simulink model "harness"  (R2023a)
settings: Solver=VariableStepAuto  StartTime=0.0  StopTime=90  FixedStep=0.001  RelTol=1e-3  EnableMultiTasking=on
model workspace (MAT data in the model file):
  c = Simulink.Parameter
  c.Value = 1500
  c.DataType = 'double'
  c.DocUnits = 'Ns/m'
  c.Complexity = 'real'
  c.Dimensions = [1 1]
  k1 = Simulink.Parameter
  k1.Value = 29000
  k1.DataType = 'double'
  k1.DocUnits = 'N/m'
  k1.Complexity = 'real'
  k1.Dimensions = [1 1]
  k2 = Simulink.Parameter
  k2.Value = 228000
  k2.DataType = 'double'
  k2.DocUnits = 'N/m'
  k2.Complexity = 'real'
  k2.Dimensions = [1 1]
  m1 = Simulink.Parameter
  m1.Value = 380
  m1.DataType = 'double'
  m1.DocUnits = 'kg'
  m1.Complexity = 'real'
  m1.Dimensions = [1 1]
  m2 = Simulink.Parameter
  m2.Value = 31
  m2.DataType = 'double'
  m2.DocUnits = 'kg'
  m2.Complexity = 'real'
  m2.Dimensions = [1 1]
undefined symbols (not defined in the file): DiscIntNeverNeededParam
libraries: simulink x2
settings Model: Creator=david  LastModifiedBy=david
settings DebuggingCC: UnconnectedInputMsg=warning  UnconnectedOutputMsg=warning  UnconnectedLineMsg=warning
settings ModelReferenceCC: EnableRefExpFcnMdlSchedulingChecks=on
settings RTWCC: DLArmComputeVersion=19.05
settings ConfigComp: CovMetricSettings=dcwe

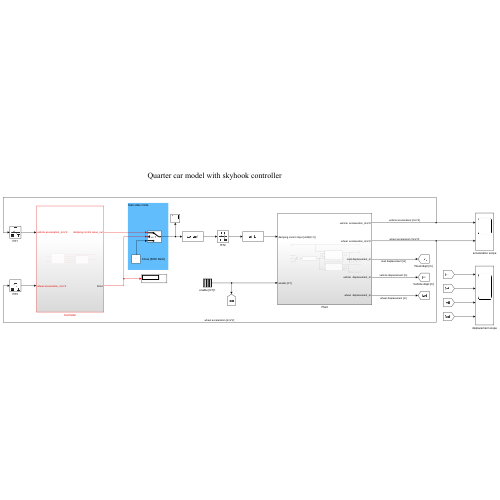
[thumbnail: Simulink's stored preview of the top-level diagram]
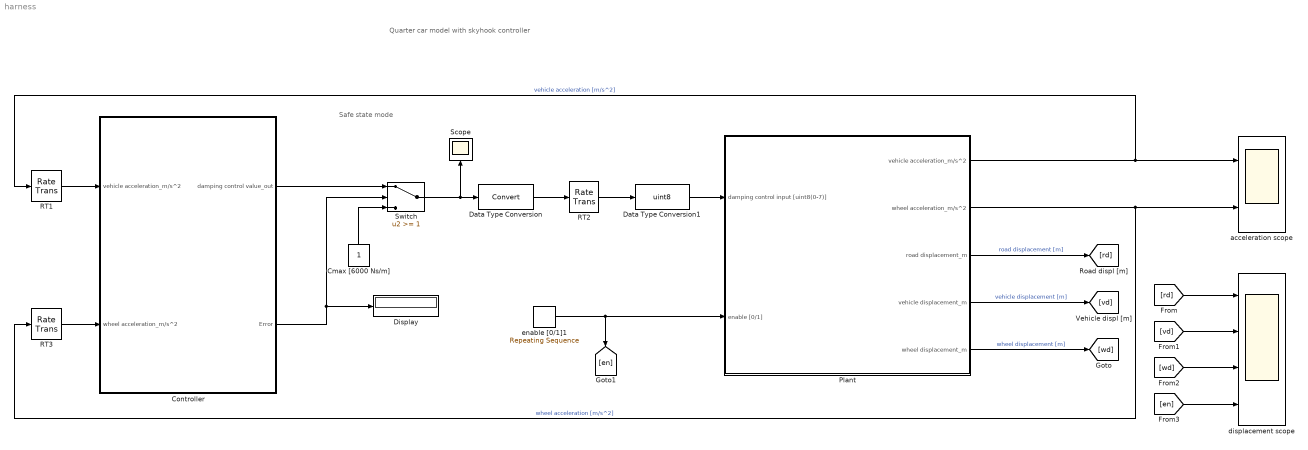
== system harness ==
  note: Safe state mode
  note: Quarter car model with skyhook controller
  Cmax [6000 Ns/m] : Constant  OutDataTypeStr=uint8
  Controller : Subsystem
  Data Type Conversion : DataTypeConversion  SaturateOnIntegerOverflow=off  RndMeth=Floor
  Data Type Conversion1 : DataTypeConversion  OutDataTypeStr=uint8  SaturateOnIntegerOverflow=off  RndMeth=Floor
  Display : Display
  Plant : Subsystem
  RT1 : RateTransition
  RT2 : RateTransition
  RT3 : RateTransition
  Scope : Scope
  Switch : Switch  Threshold=1  SaturateOnIntegerOverflow=off  InputSameDT=off
  acceleration scope : Scope  NumInputPorts=2
  displacement scope : Scope  NumInputPorts=4
  enable [0/1]1 : simulink/Sources/Repeating Sequence  rep_seq_t="[0 10  20 20.1 40 50 80 80.1]"  rep_seq_y=[0 0 0 1 1 1 1 1]
  wires:
  RT2/1 -> Data Type Conversion1/1
  Data Type Conversion1/1 -> Plant/1("damping control input [uint8(0-7)] ")
  Data Type Conversion/1 -> RT2/1
  enable [0/1]1/1 -> Plant/2(enable [0/1]), [en]
  Plant/4(vehicle displacement_m) -> [vd]  "vehicle displacement [m]"
  [wd] -> displacement scope/3
  [en] -> displacement scope/4
  Plant/5(wheel displacement_m) -> [wd]  "wheel displacement [m]"
  [rd] -> displacement scope/1
  Plant/1(vehicle acceleration_m/s^2) -> RT1/1, acceleration scope/1  "vehicle acceleration [m/s^2]"
  Plant/3(road displacement_m) -> [rd]  "road displacement [m]"
  [vd] -> displacement scope/2
  Plant/2(wheel acceleration_m/s^2) -> acceleration scope/2, RT3/1  "wheel acceleration [m/s^2]"
  Controller/1(damping control value_out) -> Switch/1
  RT1/1 -> Controller/1(vehicle acceleration_m/s^2)
  RT3/1 -> Controller/2(wheel acceleration_m/s^2)
  Controller/2(Error) -> Switch/2, Display/1
  Cmax [6000 Ns/m]/1 -> Switch/3
  Switch/1 -> Data Type Conversion/1, Scope/1

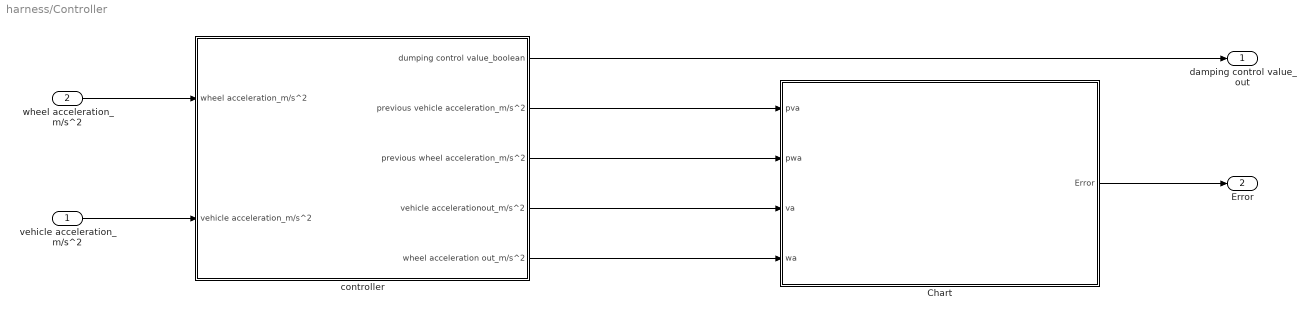
== system harness/Controller ==
  vehicle acceleration_m/s^2 : Inport  OutDataTypeStr=double  Unit=m/s^2  PortDimensions=1
  wheel acceleration_m/s^2 : Inport  Port=2  OutDataTypeStr=double  Unit=m/s^2  PortDimensions=1
  Chart : Stateflow chart  TreatAsAtomicUnit=on
  controller : Subsystem
  damping control value_out : Outport  OutDataTypeStr=uint8  PortDimensions=1  VectorParamsAs1DForOutWhenUnconnected=off
  Error : Outport  Port=2
  wires:
  vehicle acceleration_m/s^2/1 -> controller/2(vehicle acceleration_m/s^2)
  wheel acceleration_m/s^2/1 -> controller/1(wheel acceleration_m/s^2)
  Chart/1(Error) -> Error/1
  controller/1(dumping control value_boolean) -> damping control value_out/1
  controller/2(previous vehicle acceleration_m/s^2) -> Chart/1(pva)
  controller/3(previous wheel acceleration_m/s^2) -> Chart/2(pwa)
  controller/4(vehicle accelerationout_m/s^2) -> Chart/3(va)
  controller/5(wheel acceleration out_m/s^2) -> Chart/4(wa)

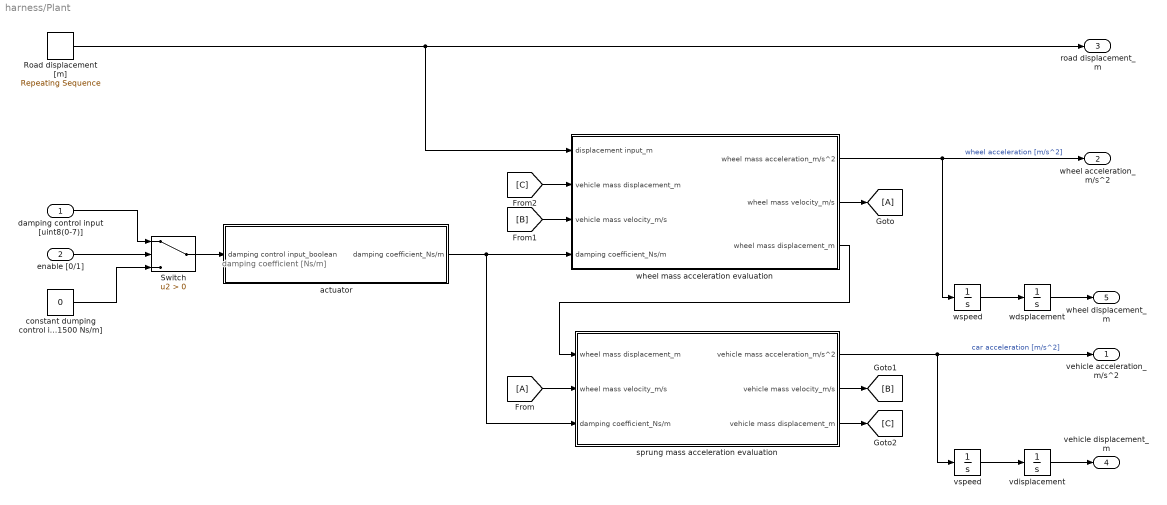
== system harness/Plant ==
  note: damping coefficient [Ns/m]
  "damping control input [uint8(0-7)] " : Inport  OutDataTypeStr=uint8
  enable [0/1] : Inport  Port=2
  From : From
  Goto : Goto
  Road displacement [m] : simulink/Sources/Repeating Sequence  rep_seq_t=[0 0.1 4 4.1 8 10 10.1 10.2 10.3 14]  rep_seq_y=[0 0.2 -0.2 0 -0.2 0 0.2 0.2 0 0]
  Switch : Switch  Criteria=u2 > Threshold  SaturateOnIntegerOverflow=off  InputSameDT=off
  actuator : Subsystem
  constant dumping control input [0=1500 Ns/m] : Constant  Value=0
  sprung mass acceleration evaluation : Subsystem
  vdisplacement : Integrator
  vspeed : Integrator
  wdsplacement : Integrator
  wheel mass acceleration evaluation : Subsystem
  wspeed : Integrator
  vehicle acceleration_m/s^2 : Outport  VectorParamsAs1DForOutWhenUnconnected=off
  wheel acceleration_m/s^2 : Outport  Port=2  Unit=m/s^2  VectorParamsAs1DForOutWhenUnconnected=off
  road displacement_m : Outport  Port=3  Unit=m  VectorParamsAs1DForOutWhenUnconnected=off
  vehicle displacement_m : Outport  Port=4  Unit=m  VectorParamsAs1DForOutWhenUnconnected=off
  wheel displacement_m : Outport  Port=5  Unit=m  VectorParamsAs1DForOutWhenUnconnected=off
  wires:
  Switch/1 -> actuator/1("damping control input_boolean ")
  actuator/1(damping coefficient_Ns/m) -> sprung mass acceleration evaluation/3(damping coefficient_Ns/m), wheel mass acceleration evaluation/4(damping coefficient_Ns/m)
  wheel mass acceleration evaluation/1(wheel mass acceleration_m/s^2) -> wheel acceleration_m/s^2/1, wspeed/1  "wheel acceleration [m/s^2]"
  wheel mass acceleration evaluation/2(wheel mass velocity_m/s) -> Goto/1
  sprung mass acceleration evaluation/1(vehicle mass acceleration_m/s^2) -> vehicle acceleration_m/s^2/1, vspeed/1  "car acceleration [m/s^2]"
  sprung mass acceleration evaluation/2(vehicle mass velocity_m/s) -> [B]
  enable [0/1]/1 -> Switch/2
  wspeed/1 -> wdsplacement/1
  From/1 -> sprung mass acceleration evaluation/2(wheel mass velocity_m/s)
  vspeed/1 -> vdisplacement/1
  wdsplacement/1 -> wheel displacement_m/1
  constant dumping control input [0=1500 Ns/m]/1 -> Switch/3
  Road displacement [m]/1 -> road displacement_m/1, wheel mass acceleration evaluation/1(displacement input_m)
  wheel mass acceleration evaluation/3(wheel mass displacement_m) -> sprung mass acceleration evaluation/1(wheel mass displacement_m)
  "damping control input [uint8(0-7)] "/1 -> Switch/1
  vdisplacement/1 -> vehicle displacement_m/1
  [B] -> wheel mass acceleration evaluation/3(vehicle mass velocity_m/s)
  sprung mass acceleration evaluation/3(vehicle mass displacement_m) -> [C]
  [C] -> wheel mass acceleration evaluation/2(vehicle mass displacement_m)

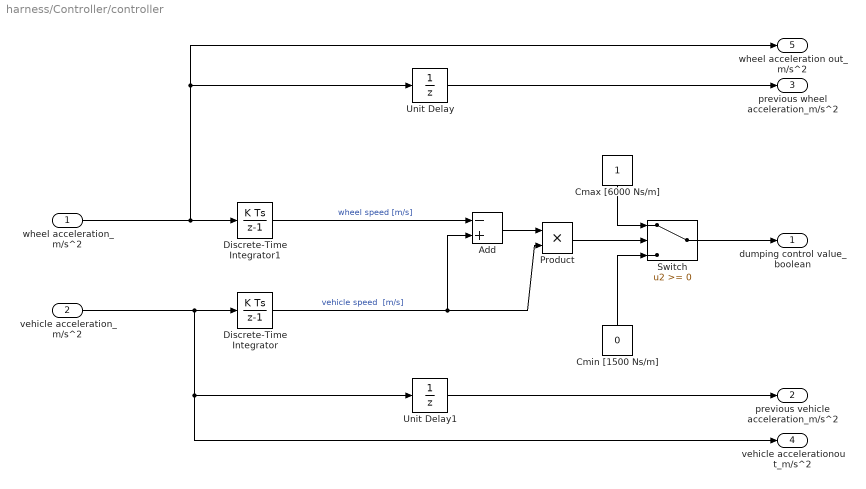
== system harness/Controller/controller ==
  wheel acceleration_m/s^2 : Inport
  vehicle acceleration_m/s^2 : Inport  Port=2  OutDataTypeStr=double  PortDimensions=1
  Add : Sum  Inputs=-+
  Cmax [6000 Ns/m] : Constant  OutDataTypeStr=uint8
  Cmin [1500 Ns/m] : Constant  Value=0  OutDataTypeStr=uint8
  Discrete-Time Integrator : DiscreteIntegrator  SampleTime=-1  ICPrevOutput=DiscIntNeverNeededParam  ICPrevScaledInput=DiscIntNeverNeededParam
  Discrete-Time Integrator1 : DiscreteIntegrator  SampleTime=-1  ICPrevOutput=DiscIntNeverNeededParam  ICPrevScaledInput=DiscIntNeverNeededParam
  Product : Product
  Switch : Switch  SaturateOnIntegerOverflow=off  InputSameDT=off
  Unit Delay : UnitDelay  SampleTime=-1  HasFrameUpgradeWarning=on
  Unit Delay1 : UnitDelay  SampleTime=-1  HasFrameUpgradeWarning=on
  dumping control value_boolean : Outport  OutDataTypeStr=uint8  VectorParamsAs1DForOutWhenUnconnected=off
  previous vehicle acceleration_m/s^2 : Outport  Port=2
  previous wheel acceleration_m/s^2 : Outport  Port=3
  vehicle accelerationout_m/s^2 : Outport  Port=4
  wheel acceleration out_m/s^2 : Outport  Port=5
  wires:
  wheel acceleration_m/s^2/1 -> wheel acceleration out_m/s^2/1, Unit Delay/1, Discrete-Time Integrator1/1
  Cmax [6000 Ns/m]/1 -> Switch/1
  Cmin [1500 Ns/m]/1 -> Switch/3
  Discrete-Time Integrator/1 -> Product/2, Add/2  "vehicle speed  [m/s]"
  Add/1 -> Product/1
  vehicle acceleration_m/s^2/1 -> vehicle accelerationout_m/s^2/1, Unit Delay1/1, Discrete-Time Integrator/1
  Product/1 -> Switch/2
  Discrete-Time Integrator1/1 -> Add/1  "wheel speed [m/s]"
  Unit Delay/1 -> previous wheel acceleration_m/s^2/1
  Unit Delay1/1 -> previous vehicle acceleration_m/s^2/1
  Switch/1 -> dumping control value_boolean/1

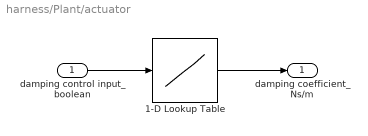
== system harness/Plant/actuator ==
  "damping control input_boolean " : Inport
  1-D Lookup Table : Lookup_n-D  NumberOfTableDimensions=1  BreakpointsForDimension1=uint8([0,1]);  Table=[1500,6000]  InternalRulePriority=Speed  RndMeth=Simplest
  damping coefficient_Ns/m : Outport  Unit=N*second/m  VectorParamsAs1DForOutWhenUnconnected=off
  wires:
  "damping control input_boolean "/1 -> 1-D Lookup Table/1
  1-D Lookup Table/1 -> damping coefficient_Ns/m/1

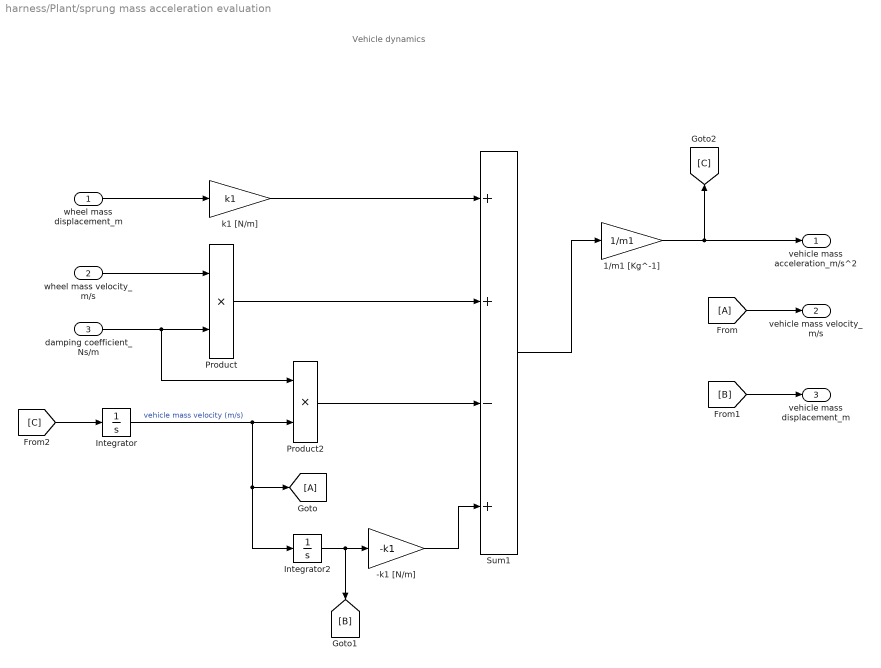
== system harness/Plant/sprung mass acceleration evaluation ==
  note: Vehicle dynamics
  wheel mass displacement_m : Inport
  wheel mass velocity_m/s : Inport  Port=2
  damping coefficient_Ns/m : Inport  Port=3  Unit=N*s/m
  -k1 [N/m] : Gain  Gain=-k1
  1/m1 [Kg^-1] : Gain  Gain=1/m1
  From : From
  Goto : Goto
  Integrator : Integrator
  Integrator2 : Integrator
  Product : Product
  Product2 : Product
  Sum1 : Sum  Inputs=++-+
  k1 [N/m] : Gain  Gain=k1
  vehicle mass acceleration_m/s^2 : Outport  Unit=m/s^2  VectorParamsAs1DForOutWhenUnconnected=off
  vehicle mass velocity_m/s : Outport  Port=2  Unit=m/s  VectorParamsAs1DForOutWhenUnconnected=off
  vehicle mass displacement_m : Outport  Port=3  Unit=m  VectorParamsAs1DForOutWhenUnconnected=off
  wires:
  Sum1/1 -> 1/m1 [Kg^-1]/1
  Integrator/1 -> Integrator2/1, Goto/1, Product2/2  "vehicle mass velocity (m/s)"
  Integrator2/1 -> [B], -k1 [N/m]/1
  wheel mass displacement_m/1 -> k1 [N/m]/1
  wheel mass velocity_m/s/1 -> Product/1
  damping coefficient_Ns/m/1 -> Product2/1, Product/2
  k1 [N/m]/1 -> Sum1/1
  Product/1 -> Sum1/2
  Product2/1 -> Sum1/3
  1/m1 [Kg^-1]/1 -> [C], vehicle mass acceleration_m/s^2/1
  -k1 [N/m]/1 -> Sum1/4
  From/1 -> vehicle mass velocity_m/s/1
  [B] -> vehicle mass displacement_m/1
  [C] -> Integrator/1

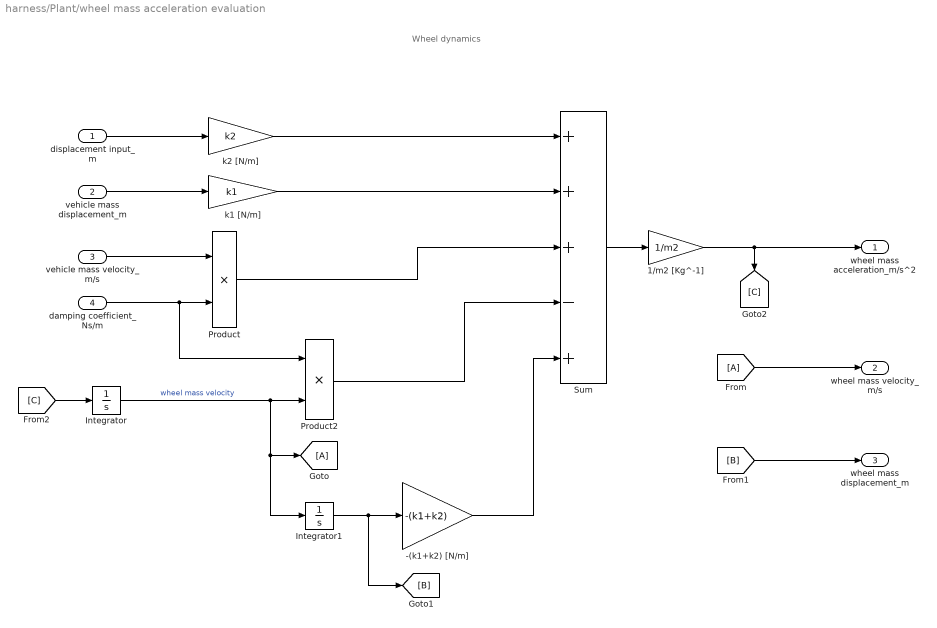
== system harness/Plant/wheel mass acceleration evaluation ==
  note: Wheel dynamics
  displacement input_m : Inport  OutDataTypeStr=double  Unit=m
  vehicle mass displacement_m : Inport  Port=2  Unit=m
  vehicle mass velocity_m/s : Inport  Port=3  Unit=m/s
  damping coefficient_Ns/m : Inport  Port=4  Unit=N*sec/m
  -(k1+k2) [N/m] : Gain  Gain=-(k1+k2)
  1/m2 [Kg^-1] : Gain  Gain=1/m2
  From : From
  Goto : Goto
  Integrator : Integrator
  Integrator1 : Integrator
  Product : Product
  Product2 : Product
  Sum : Sum  Inputs=+++-+
  k1 [N/m] : Gain  Gain=k1
  k2 [N/m] : Gain  Gain=k2
  wheel mass acceleration_m/s^2 : Outport  Unit=m/s^2  VectorParamsAs1DForOutWhenUnconnected=off
  wheel mass velocity_m/s : Outport  Port=2  Unit=m/s  VectorParamsAs1DForOutWhenUnconnected=off
  wheel mass displacement_m : Outport  Port=3  Unit=m  VectorParamsAs1DForOutWhenUnconnected=off
  wires:
  Sum/1 -> 1/m2 [Kg^-1]/1
  k2 [N/m]/1 -> Sum/1
  Integrator/1 -> Goto/1, Integrator1/1, Product2/2  "wheel mass velocity"
  Integrator1/1 -> [B], -(k1+k2) [N/m]/1
  vehicle mass displacement_m/1 -> k1 [N/m]/1
  displacement input_m/1 -> k2 [N/m]/1
  vehicle mass velocity_m/s/1 -> Product/1
  damping coefficient_Ns/m/1 -> Product2/1, Product/2
  k1 [N/m]/1 -> Sum/2
  Product/1 -> Sum/3
  Product2/1 -> Sum/4
  -(k1+k2) [N/m]/1 -> Sum/5
  1/m2 [Kg^-1]/1 -> wheel mass acceleration_m/s^2/1, [C]
  From/1 -> wheel mass velocity_m/s/1
  [B] -> wheel mass displacement_m/1
  [C] -> Integrator/1

== stateflow chart harness/Controller/Chart ==
  state ErrorLogic
    state NO_ERROR
      en:
      Error=0;
    state CHECK_STATE
    state ERROR
      en:
      Error=1
    (default) -> NO_ERROR
    NO_ERROR -> CHECK_STATE
    CHECK_STATE -> ERROR [order 1] : after(20,msec)
    CHECK_STATE -> NO_ERROR [order 2] : [(va) ~= (pva) && (wa) ~= (pwa)]
  data: pva input double; pwa input double; va input double; wa input double; Error output uint8
